simulink model "power_simulation2022a"  (R2022a)
settings: Solver=VariableStepAuto  StartTime=0.0  StopTime=600  RelTol=1e-3
values from neighbouring files (symbols this model uses):
  Ts = 5E-6    (= 5e-06)    [motor_variables.m]
undefined symbols (not defined in the file or in its folder): g_ft, sigbuilder_block
libraries: fl_lib x21, nesl_utility x11, ee_lib x4, sdl_lib x2
settings Model: Creator=OADEBAJO  LastModifiedBy=OADEBAJO

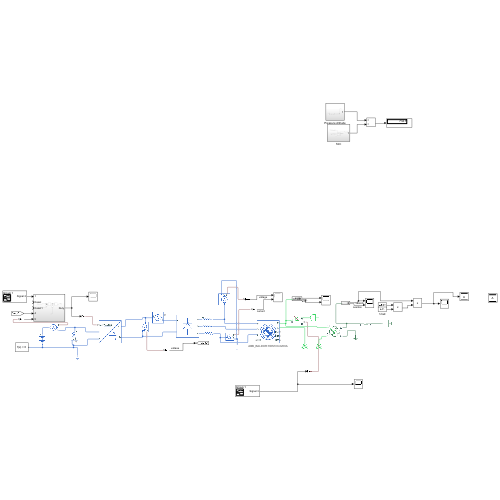
[thumbnail: Simulink's stored preview of the top-level diagram]
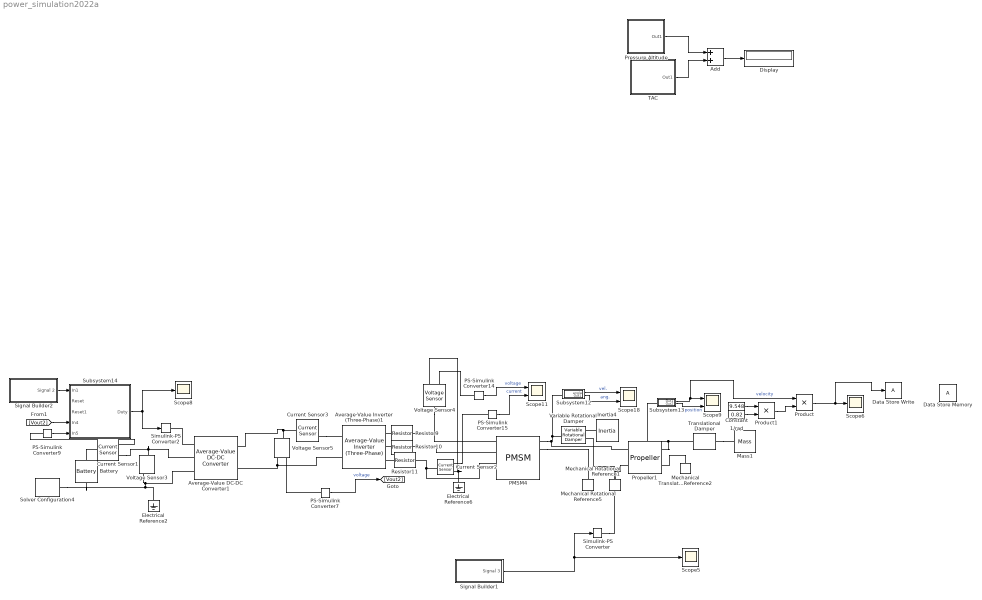
== system power_simulation2022a ==
  1/rad : Constant  Value=0.82
  Add : Sum
  Average-Value Inverter (Three-Phase)1 : ee_lib/Semiconductors & Converters/Converters/Average-Value Inverter (Three-Phase)  port_option=ee.enum.threePhasePort.expanded  FRated=60 Hz  PhaseShift=60 deg  voltage_ratio=sqrt(6) / pi  Pfixed=1e3 W  v_on=100 V  v_off=75 V
      settings: SourceProductBaseCode=PS  InternalSimscapePortConfiguration="{\"Bottom\":[],\"Left\":[{\"id\":\"p\",\"label\":\"+\",\"type\":\"foundation.electrical.electrical\"},{\"id\":\"n\",\"label\":\"-\",\"type\":\"foundation.electrical.electrical\"}],\"Right\":[{\"id\":\"a\",\"label\":\"a\",\"type\":\"foundation.electrical.electrical\"},{\"id\":\"b\",\"label\":\"b\",\"type\":\"foundation.electrical.electrical\"},{\"id\":\"c\",\"label\":\"c\",\"type\":\"foundation.electrical.electrical\"}],\"Top\":[]}"
  Average-Value DC-DC Converter1 : ee_lib/Semiconductors & Converters/Converters/Average-Value DC-DC Converter  control_option=ee.enum.converters.controlinput.dutycycle  converter_type=ee.enum.converters.dcdctype.buckboost  efficiency_option=ee.enum.converters.efficiency.constant  efficiency_fixed=95  i_vec=[0, 2, 5] A  efficiency_vec=[90, 95, 98]
      settings: SourceProductBaseCode=PS  InternalSimscapePortConfiguration="{\"Bottom\":[],\"Left\":[{\"id\":\"DutyCycle\",\"label\":\"DutyCycle\",\"type\":\"input\"},{\"id\":\"p1\",\"label\":\"1+\",\"type\":\"foundation.electrical.electrical\"},{\"id\":\"n1\",\"label\":\"1-\",\"type\":\"foundation.electrical.electrical\"}],\"Right\":[{\"id\":\"p2\",\"label\":\"2+\",\"type\":\"foundation.electrical.electrical\"},{\"id\":\"n2\",\"label\":\"2-\",\"type\":\"foundation.electrical.electrical\"}],\"Top\":[]}"
  Battery : ee_lib/Sources/Battery  Vnom=300 V  prm_dir=ee.enum.batterybasic.prm_dir.disabled  R1_dis=2 Ohm  R1_ch=2 Ohm  R1=0.001 Ohm  prm_AH=ee.enum.batterybasic.prm_AH.finite  AH=50 A*hr  V1=11.5 V  AH1=25 A*hr  prm_R2=ee.enum.batterybasic.prm_R2.disabled  R2=2000 Ohm  prm_dyn=ee.enum.batterybasic.prm_dyn.off  Rp1=0.005 Ohm  tau1=30 s  Rp2=0.005 Ohm  tau2=30 s  Rp3=0.005 Ohm  tau3=30 s  Rp4=0.005 Ohm  tau4=30 s  Rp5=0.005 Ohm  tau5=30 s  prm_fade=ee.enum.batterybasic.prm_fade.disabled  N_fade=100  AH_fade=45 A*hr  R1_fade=2.02 Ohm  R1_ch_fade=2.02 Ohm  V1_fade=10.35 V  prm_age=ee.enum.batterybasic.prm_age.disabled  prm_age_OCV=ee.enum.batterybasic.prm_age_OCV.OCV  OCV_age=0.9  SOC_age=60  delta_time_age_vec=[0] d  temperature_age_vec=[273] K  OCV_scaling_age=2.2134e6  OCV_offset_age=1.632e6  temp_exp_age=0.515833569 V  t_exp_age=0.75  i_specify=off  i_priority=None  i=0 A  i_nominal_specify=off  i_nominal_unit=A  i_nominal_value=1  v_specify=off  v_priority=None  v=0 V  v_nominal_specify=off  v_nominal_unit=V  v_nominal_value=1  charge_specify=off  charge_priority=High  charge=50 A*hr  charge_nominal_specify=off  charge_nominal_unit=A*hr  charge_nominal_value=1  num_cycles_specify=off  num_cycles_priority=High  num_cycles=0  num_cycles_nominal_specify=off  num_cycles_nominal_unit=1  num_cycles_nominal_value=1  Tmeas=298.15 K  Tmeas_age=298.15 K  Vnom_T2=12 V  R1_T2=2.2 Ohm  R1_T2_dis=2.2 Ohm  R1_T2_ch=2.2 Ohm  V1_T2=11.4 V  R2_T2=2200 Ohm  Rp1_T2=0.005 Ohm  tau1_T2=30 s  Rp2_T2=0.005 Ohm  tau2_T2=30 s  Rp3_T2=0.005 Ohm  tau3_T2=30 s  Rp4_T2=0.005 Ohm  tau4_T2=30 s  Rp5_T2=0.005 Ohm  tau5_T2=30 s  Tmeas2=273.15 K  thermal_mass=30000 J/K  temperature_specify=off  temperature_priority=High  temperature=298.15 K  temperature_nominal_specify=off  temperature_nominal_unit=K  temperature_nominal_value=1
  Constant : Constant  Value=9.548
  Current Sensor1 : fl_lib/Electrical/Electrical Sensors/Current Sensor
      settings: SourceProductBaseCode=PW,SS,VE
  Current Sensor2 : fl_lib/Electrical/Electrical Sensors/Current Sensor
      settings: SourceProductBaseCode=PW,SS,VE
  Current Sensor3 : fl_lib/Electrical/Electrical Sensors/Current Sensor
      settings: SourceProductBaseCode=PW,SS,VE
  Data Store Memory : DataStoreMemory  WriteAfterWriteMsg=warning  ShowAdditionalParam=off
  Data Store Write : DataStoreWrite  IndexOptions=Index vector (dialog)  Indices=1  OutputSizes=1
  Display : Display
  Electrical Reference2 : fl_lib/Electrical/Electrical Elements/Electrical Reference
      settings: SourceProductBaseCode=PW,SS,VE
  Electrical Reference6 : fl_lib/Electrical/Electrical Elements/Electrical Reference
      settings: SourceProductBaseCode=PW,SS,VE
  Inertia4 : fl_lib/Mechanical/Rotational Elements/Inertia  inertia=0.01 kg*m^2  num_ports=foundation.enum.numPorts2.one  w_specify=off  w_priority=High  w=0 rad/s  w_nominal_specify=off  w_nominal_unit=rad/s  w_nominal_value=1  t_specify=off  t_priority=None  t=0 N*m  t_nominal_specify=off  t_nominal_unit=N*m  t_nominal_value=1
      settings: SourceProductBaseCode=PW,SS,VE
  Mass1 : fl_lib/Mechanical/Translational Elements/Mass  mass=6 kg  num_ports=foundation.enum.numPorts2.one  v_specify=off  v_priority=High  v=0 m/s  v_nominal_specify=off  v_nominal_unit=m/s  v_nominal_value=1  f_specify=off  f_priority=None  f=0 N  f_nominal_specify=off  f_nominal_unit=N  f_nominal_value=1
      settings: SourceProductBaseCode=PW,SS,VE
  Mechanical Rotational Reference1 : fl_lib/Mechanical/Rotational Elements/Mechanical Rotational Reference
      settings: SourceProductBaseCode=PW,SS,VE
  Mechanical Rotational Reference5 : fl_lib/Mechanical/Rotational Elements/Mechanical Rotational Reference
      settings: SourceProductBaseCode=PW,SS,VE
  Mechanical Translational Reference2 : fl_lib/Mechanical/Translational Elements/Mechanical Translational Reference
      settings: SourceProductBaseCode=PW,SS,VE
  PMSM4 : ee_lib/Electromechanical/Permanent Magnet/PMSM  Tag={'toolbox/physmod/elec/library/m/ee_lib_parts';'Electromechanical/Permanent_Magnet/PMSM/ABB_BALDOR/HDS100_0206A.xml'}  port_option=ee.enum.threePhasePort.expanded  winding_type=ee.enum.statorconnection.wye  machine_param=ee.enum.pmsm.parameterization.constant  nPolePairs=5  pmflux_param=ee.enum.pmflux.fluxlinkage  pm_flux_linkage=0.0686133185085635 Wb  torque_constant=0.343066592542818 N*m/A  back_emf_constant=0.343066592542818 V/(rad/s)  stator_param=ee.enum.statorparam.LdLqL0  Ld=0.00855 H  Lq=0.00855 H  idVec=[-200 0 200] % Parameter not set A  iqVec=[-200 0 200] % Parameter not set A  LdMatrix=[0.0002 0.0002 0.0002;0.0002 0.0002 0.0002;0.0002 0.0002 0.0002] % Parameter not set H  LqMatrix=[0.0002 0.0002 0.0002;0.0002 0.0002 0.0002;0.0002 0.0002 0.0002] % Parameter not set H  PmMatrix=[0.1 0.1 0.1;0.1 0.1 0.1;0.1 0.1 0.1] Wb  ktMatrix=[0.18 0.18 0.18;0.18 0.18 0.18;0.18 0.18 0.18] N*m/A  keMatrix=[0.18 0.18 0.18;0.18 0.18 0.18;0.18 0.18 0.18] % Parameter not set V/(rad/s)  L0=[] % Parameter not set H  Ls=0.0002 H  Lm=-2e-05 H  Ms=2e-05 H  Rs=1.46 Ohm  zero_sequence=ee.enum.park.zerosequence.exclude  axes_param=ee.enum.rotorangle.daxis  loss_param=ee.enum.ironloss.none  losses_oc=[0 0 0] % Parameter not set W  losses_sc=[0 0 0] % Parameter not set W  f_losses=60 % Parameter not set Hz  Isc_losses=95 % Parameter not set A  J=7.6e-05 kg*m^2  lam=0 % Parameter not set N*m/(rad/s)  i_d_specify=off  i_d_priority=None  i_d=0 A  i_d_nominal_specify=off  i_d_nominal_unit=A  i_d_nominal_value=1  i_q_specify=off  i_q_priority=None  i_q=0 A  i_q_nominal_specify=off  i_q_nominal_unit=A  i_q_nominal_value=1  torque_specify=off  torque_priority=None  torque=0 N*m  torque_nominal_specify=off  torque_nominal_unit=N*m  torque_nominal_value=1  angular_velocity_specify=off  angular_velocity_priority=High  angular_velocity=0 rpm  angular_velocity_nominal_specify=off  angular_velocity_nominal_unit=rpm  angular_velocity_nominal_value=1  angular_position_specify=off  angular_position_priority=High  angular_position=0 deg  angular_position_nominal_specify=off  angular_position_nominal_unit=deg  angular_position_nominal_value=1  alpha=3.93e-3 1/K  alpha_flux=-0.001 1/K  Tmeas=298.15 K  stator_thermal_mass=100 J/K  rotor_thermal_mass=200 J/K  Rm_percent_rotor=90  Rd_percent_rotor=30  temperatureA_specify=off  temperatureA_priority=High  temperatureA=25 degC  temperatureA_nominal_specify=off  temperatureA_nominal_unit=degC  temperatureA_nominal_value=1  temperatureB_specify=off  temperatureB_priority=High  temperatureB=25 degC  temperatureB_nominal_specify=off  temperatureB_nominal_unit=degC  temperatureB_nominal_value=1  temperatureC_specify=off  temperatureC_priority=High  temperatureC=25 degC  temperatureC_nominal_specify=off  temperatureC_nominal_unit=degC  temperatureC_nominal_value=1  temperatureR_specify=off  temperatureR_priority=High  temperatureR=25 degC  temperatureR_nominal_specify=off  temperatureR_nominal_unit=degC  temperatureR_nominal_value=1
      settings: AttributesFormatString=ABB_BALDOR:HDS100-0206A  InternalSimscapePortConfiguration="{\"Bottom\":[],\"Left\":[{\"id\":\"a\",\"label\":\"a\",\"type\":\"foundation.electrical.electrical\"},{\"id\":\"b\",\"label\":\"b\",\"type\":\"foundation.electrical.electrical\"},{\"id\":\"c\",\"label\":\"c\",\"type\":\"foundation.electrical.electrical\"},{\"id\":\"HR\",\"label\":\"HR\",\"type\":\"foundation.thermal.thermal\"}],\"Right\":[{\"id\":\"R\",\"label\":\"R\",\"type\":\"foundation.mechanical.rotational.rotational\"},{\"id\":\"C\",\"label\":\"C\",\"type\":\"foundation.mechanical.rotational.rotational\"},{\"id\":\"HA\",\"label\":\"HA\",\"type\":\"foundation.thermal.thermal\"},{\"id\":\"HB\",\"label\":\"HB\",\"type\":\"foundation.thermal.thermal\"},{\"id\":\"HC\",\"label\":\"HC\",\"type\":\"foundation.thermal.thermal\"}],\"Top\":[]}"
  PS-Simulink Converter14 : nesl_utility/PS-Simulink Converter  PhysicalDomain=network_engine_domain  SubClassName=ps_output  LeftPortType=input  RightPortType=output  PseudoPeriodic=off  Frequencies=[]  VectorFormat=inherit  Unit=inherit  AffineConversion=off
      settings: SourceProductBaseCode=SS,PW,VE
  PS-Simulink Converter15 : nesl_utility/PS-Simulink Converter  PhysicalDomain=network_engine_domain  SubClassName=ps_output  LeftPortType=input  RightPortType=output  PseudoPeriodic=off  Frequencies=[]  VectorFormat=inherit  Unit=inherit  AffineConversion=off
      settings: SourceProductBaseCode=SS,PW,VE
  PS-Simulink Converter7 : nesl_utility/PS-Simulink Converter  PhysicalDomain=network_engine_domain  SubClassName=ps_output  LeftPortType=input  RightPortType=output  PseudoPeriodic=off  Frequencies=[]  VectorFormat=inherit  Unit=inherit  AffineConversion=off
      settings: SourceProductBaseCode=SS,PW,VE
  PS-Simulink Converter9 : nesl_utility/PS-Simulink Converter  PhysicalDomain=network_engine_domain  SubClassName=ps_output  LeftPortType=input  RightPortType=output  PseudoPeriodic=off  Frequencies=[]  VectorFormat=1-D array  Unit=A  AffineConversion=off
      settings: SourceProductBaseCode=SS,PW,VE
  Pressure Altitude : Subsystem
  Product : Product
  Product1 : Product
  Propeller1 : sdl_lib/Engines & Motors/Propeller  parameterization=sdl.enum.PropellerParameterization.Constant  pitch_type=foundation.enum.constant_controlled.constant  D=0.2 m  kt_const=0.25  kq_const=0.05  kt_poly_fixed=[.063, -.19, -.25, .37]  kq_poly_fixed=[.0043, -.021, -.03, .05]  pitch_ratio_TLU=[-.5, .5, .7, .9, 1.1, 1.4]  kt_poly_TLU=[.04, -.1, -.24, .12; .118, -.24, -.24, .19; .082, -.21, -.25, .28; .063, -.19, -.25, .37; .055, -.17, -.25, .45; .064, -.21, -.19, .55]  kq_poly_TLU=[.02, -.06, -.02, .02; .04, -.034, -.016, .018; .0076, -.02, -.023, .031; .0043, -.021, -.03, .05; .0047, -.024, -.036, .073; .0045, -.025, -.044, .11]  J_tab_TLU=[0, .3, .5, .7, .9, 1.2, 1.5]  kt_tab_fixed=[.37, .28, .21, .12, .033, -.098, -.23]  kq_tab_fixed=[.049, .039, .03, .02, .0096, -.0093, -.028]  kt_tab_TLU=[.12, .04, -.02, -.083, -.15, -.24, -.33; .19, .1, .029, -.047, -.12, -.23, -.35; .28, .19, .12, .032, -.054, -.18, -.31; .37, .28, .21, .12, .033, -.098, -.23; .45, .36, .29, .21, .13, -.0057, -.16; .54, .47, .41, .33, .25, .13, .0029]  kq_tab_TLU=[.02, .0091, -.0025, -.017, -.032, -.056, -.078; .017, .011, .006, .0009, -.0041, -.012, -.019; .03, .022, .015, .0074, -.0008, -.013, -.026; .049, .039, .03, .02, .0096, -.0093, -.028; .072, .06, .05, .038, .025, .0042, -.015; .11, .097, .085, .071, .057, .033, .0065]  interp_method=simscape.enum.interpolation.linear  extrap_method=simscape.enum.extrapolation.linear  density_spec=foundation.enum.constant_variable.constant  rho=1000 kg/m^3  translational_ports=sdl.enum.ConnectionType.Conserving  wake_fraction=0.2  efficiency_sensor=simscape.enum.onoff.off  n_thr=0.001 Hz  k_thr=0.001  operation_check=simscape.enum.assert.action.warn  w_specify=off  w_priority=None  w=0 rad/s  w_nominal_specify=off  w_nominal_unit=rad/s  w_nominal_value=1  Q_specify=off  Q_priority=None  Q=0 N*m  Q_nominal_specify=off  Q_nominal_unit=N*m  Q_nominal_value=1  v_specify=off  v_priority=None  v=0 m/s  v_nominal_specify=off  v_nominal_unit=m/s  v_nominal_value=1  thrust_specify=off  thrust_priority=None  thrust=0 N  thrust_nominal_specify=off  thrust_nominal_unit=N  thrust_nominal_value=1
      settings: SourceProductBaseCode=LD  InternalSimscapePortConfiguration="{\"Bottom\":[],\"Left\":[{\"id\":\"R1\",\"label\":\"R1\",\"type\":\"foundation.mechanical.rotational.rotational\"},{\"id\":\"C1\",\"label\":\"C1\",\"type\":\"foundation.mechanical.rotational.rotational\"}],\"Right\":[{\"id\":\"R2\",\"label\":\"R2\",\"type\":\"foundation.mechanical.translational.translational\"},{\"id\":\"C2\",\"label\":\"C2\",\"type\":\"foundation.mechanical.translational.translational\"}],\"Top\":[]}"
  Resistor10 : fl_lib/Electrical/Electrical Elements/Resistor  R=10 Ohm  i_specify=off  i_priority=None  i=0 A  i_nominal_specify=off  i_nominal_unit=A  i_nominal_value=1  v_specify=off  v_priority=None  v=0 V  v_nominal_specify=off  v_nominal_unit=V  v_nominal_value=1
      settings: SourceProductBaseCode=PW,SS,VE
  Resistor11 : fl_lib/Electrical/Electrical Elements/Resistor  R=10 Ohm  i_specify=off  i_priority=None  i=0 A  i_nominal_specify=off  i_nominal_unit=A  i_nominal_value=1  v_specify=off  v_priority=None  v=0 V  v_nominal_specify=off  v_nominal_unit=V  v_nominal_value=1
      settings: SourceProductBaseCode=PW,SS,VE
  Resistor9 : fl_lib/Electrical/Electrical Elements/Resistor  R=10 Ohm  i_specify=off  i_priority=None  i=0 A  i_nominal_specify=off  i_nominal_unit=A  i_nominal_value=1  v_specify=off  v_priority=None  v=0 V  v_nominal_specify=off  v_nominal_unit=V  v_nominal_value=1
      settings: SourceProductBaseCode=PW,SS,VE
  Scope11 : Scope  NumInputPorts=2
  Scope18 : Scope  NumInputPorts=2
  Scope5 : Scope
  Scope6 : Scope
  Scope8 : Scope
  Scope9 : Scope  NumInputPorts=2
  Signal Builder1 : Subsystem  Tag=STV Subsys  LoadFcn=sigbuilder_block('load');  StartFcn=sigbuilder_block('start');  StopFcn=sigbuilder_block('stop');  ClipboardFcn=sigbuilder_block('clipboard');  mask(Sigbuilder block){tuvar=[0:10]}
      mask help: Simulink:masks:SigbuilderBlock_MD
      mask init:
      | if ~strcmp(get_param(bdroot(gcbh),'SimulationStatus'),'stopped') tuvar = sigbuilder_block('maskInit'); end
      settings: CopyFcn=sigbuilder_block('copy');  DeleteFcn=sigbuilder_block('delete');  ModelCloseFcn=sigbuilder_block('modelClose');  PreSaveFcn=sigbuilder_block('preSave');  PauseFcn=sigbuilder_block('pause');  ContinueFcn=sigbuilder_block('continue');  NameChangeFcn=sigbuilder_block('namechange');  OpenFcn=sigbuilder_block('open',[255.75 99 836.25 501.75 ]);  CloseFcn=sigbuilder_block('close');
      mask Display: plot(0, 0, 100, 100,[2, 2, 32, 32, 2], [68, 8, 8, 68, 68],[32, 2], [38, 38], [32, 19, 2],[53, 60, 44], [32, 17, 17, 2],[16, 16, 31, 31]);txt = getActiveGroup(gcbh);text(2, 100, txt,'verticalAlignment', 'top');
  Signal Builder2 : Subsystem  Tag=STV Subsys  LoadFcn=sigbuilder_block('load');  StartFcn=sigbuilder_block('start');  StopFcn=sigbuilder_block('stop');  ClipboardFcn=sigbuilder_block('clipboard');  mask(Sigbuilder block){tuvar=[0:10]}
      mask help: Simulink:masks:SigbuilderBlock_MD
      mask init:
      | if ~strcmp(get_param(bdroot(gcbh),'SimulationStatus'),'stopped') tuvar = sigbuilder_block('maskInit'); end
      settings: CopyFcn=sigbuilder_block('copy');  DeleteFcn=sigbuilder_block('delete');  ModelCloseFcn=sigbuilder_block('modelClose');  PreSaveFcn=sigbuilder_block('preSave');  PauseFcn=sigbuilder_block('pause');  ContinueFcn=sigbuilder_block('continue');  NameChangeFcn=sigbuilder_block('namechange');  OpenFcn=sigbuilder_block('open',[255.75 99 836.25 501.75 ]);  CloseFcn=sigbuilder_block('close');
      mask Display: plot(0, 0, 100, 100,[2, 2, 32, 32, 2], [68, 8, 8, 68, 68],[32, 2], [38, 38], [32, 19, 2],[53, 60, 44], [32, 17, 17, 2],[16, 16, 31, 31]);txt = getActiveGroup(gcbh);text(2, 100, txt,'verticalAlignment', 'top');
  Simulink-PS Converter : nesl_utility/Simulink-PS Converter  PhysicalDomain=network_engine_domain  SubClassName=ps_input  LeftPortType=input  RightPortType=output  PseudoPeriodic=off  Frequencies=[]  NoiseDistribution=none  NoiseParameters=[]  Unit=1  AffineConversion=off  FilteringAndDerivatives=provide  SimscapeFilterOrder=1  InputFilterTimeConstant=0.001  UdotUserProvided=0
      settings: SourceProductBaseCode=SS,PW,VE
  Simulink-PS Converter2 : nesl_utility/Simulink-PS Converter  PhysicalDomain=network_engine_domain  SubClassName=ps_input  LeftPortType=input  RightPortType=output  PseudoPeriodic=off  Frequencies=[]  NoiseDistribution=none  NoiseParameters=[]  Unit=1  AffineConversion=off  FilteringAndDerivatives=provide  SimscapeFilterOrder=1  InputFilterTimeConstant=0.001  UdotUserProvided=0
      settings: SourceProductBaseCode=SS,PW,VE
  Solver Configuration4 : nesl_utility/Solver Configuration  PhysicalDomain=network_engine_domain  SubClassName=solver  LeftPortType=input  RightPortType=generic  Tones=[]  Harmonics=[]  SimulateNoise=off  Profile=off  UseLocalSampling=off  EnableSwitchedLinearOptims=on  FrequencyDomain=off  UseCCode=off  RelTol=0.001  AbsTol=1e-06  MinStep=1e-09  ToWorkspace=off  RevertToSquareIcSolve=off  NumHomotopyIterations=100  PhasorMode=off  PhasorModeNumHarmonics=1  IndexReductionMethod=DerivativeReplacement  DoDC=off  ResidualTolerance=1e-3  UseLocalSolver=on  LocalSolverChoice=NE_BACKWARD_EULER_ADVANCER  LocalSolverSampleTime=1e-4  DoFixedCost=on  MaxNonlinIter=3  MaxModeIter=2  ComputeImpulses=off  ImpulseIterations=2  LinearAlgebra=auto  LinearAlgebraNumThread=0  EquationFormulation=NE_TIME_EF  DelaysMemoryBudget=1024  AutomaticFiltering=off  FilteringTimeConstant=0.001  PartitionStorageMethod=AS_NEEDED  PartitionMemoryBudget=1024  PartitionMethod=FAST
      settings: SourceProductBaseCode=SS,PW,VE
  Subsystem12 : Subsystem
  Subsystem13 : Subsystem
  Subsystem14 : Subsystem
  TAC : Subsystem
  Translational Damper : fl_lib/Mechanical/Translational Elements/Translational Damper  D=100 N*s/m  v_specify=off  v_priority=None  v=0 m/s  v_nominal_specify=off  v_nominal_unit=m/s  v_nominal_value=1  f_specify=off  f_priority=None  f=0 N  f_nominal_specify=off  f_nominal_unit=N  f_nominal_value=1
      settings: SourceProductBaseCode=PW,SS,VE
  Variable Rotational Damper : sdl_lib/Couplings & Drives/Springs & Dampers/Variable Rotational Damper  Bmin=0 N*m*s/rad
      settings: SourceProductBaseCode=LD  InternalSimscapePortConfiguration="{\"Bottom\":[],\"Left\":[{\"id\":\"B\",\"label\":\"B\",\"type\":\"input\"},{\"id\":\"R\",\"label\":\"R\",\"type\":\"foundation.mechanical.rotational.rotational\"}],\"Right\":[{\"id\":\"C\",\"label\":\"C\",\"type\":\"foundation.mechanical.rotational.rotational\"}],\"Top\":[]}"
  Voltage Sensor3 : fl_lib/Electrical/Electrical Sensors/Voltage Sensor
      settings: SourceProductBaseCode=PW,SS,VE
  Voltage Sensor4 : fl_lib/Electrical/Electrical Sensors/Voltage Sensor
      settings: SourceProductBaseCode=PW,SS,VE
  Voltage Sensor5 : fl_lib/Electrical/Electrical Sensors/Voltage Sensor
      settings: SourceProductBaseCode=PW,SS,VE
  wires:
  Pressure Altitude/1(Out1) -> Add/1
  TAC/1(Out1) -> Add/2
  Add/1 -> Display/1
  PS-Simulink Converter7/1 -> [Vout2]  "voltage"
  [Vout2] -> Subsystem14/4(In4)
  Subsystem12/1(angle) -> Scope18/1  "vel."
  PS-Simulink Converter9/1 -> Subsystem14/5(In5)
  Subsystem12/2(Out1) -> Scope18/2  "ang."
  Subsystem14/1(Duty) -> Simulink-PS Converter2/1, Scope8/1
  Subsystem13/2(Out2) -> Scope9/2  "position"
  Subsystem13/1(Out1) -> Product/1, Scope9/1  "velocity"
  Signal Builder2/1(Signal 2) -> Subsystem14/1(In1)
  Signal Builder1/1(Signal 3) -> Simulink-PS Converter/1, Scope5/1
  Constant/1 -> Product1/1
  1/rad/1 -> Product1/2
  Product1/1 -> Product/2
  Product/1 -> Data Store Write/1, Scope6/1
  PS-Simulink Converter14/1 -> Scope11/1  "voltage"
  PS-Simulink Converter15/1 -> Scope11/2  "current"
  connections:
  Voltage Sensor3/RConn2 -- Average-Value DC-DC Converter1/LConn3 -- Electrical Reference2/LConn1 -- Battery/RConn1 -- Solver Configuration4/RConn1
  PMSM4/RConn1 -- Propeller1/LConn1 -- Variable Rotational Damper/RConn1 -- Subsystem12/LConn1
  Translational Damper/RConn1 -- Propeller1/RConn1 -- Subsystem13/LConn1
  Current Sensor1/RConn2 -- Average-Value DC-DC Converter1/LConn2 -- Voltage Sensor3/LConn1
  Current Sensor3/LConn1 -- Average-Value DC-DC Converter1/RConn1 -- Voltage Sensor5/LConn1
  Average-Value Inverter (Three-Phase)1/LConn2 -- Average-Value DC-DC Converter1/RConn2 -- Voltage Sensor5/RConn2
  Simulink-PS Converter/RConn1 -- Variable Rotational Damper/LConn1
  Average-Value Inverter (Three-Phase)1/RConn3 -- Resistor11/LConn1
  Resistor10/RConn1 -- PMSM4/LConn2
  Current Sensor1/LConn1 -- Battery/LConn1
  PS-Simulink Converter9/LConn1 -- Current Sensor1/RConn1
  Translational Damper/LConn1 -- Mass1/LConn1
  Average-Value DC-DC Converter1/LConn1 -- Simulink-PS Converter2/RConn1
  Current Sensor2/LConn1 -- Resistor11/RConn1 -- PMSM4/LConn3
  Resistor9/RConn1 -- Voltage Sensor4/LConn1 -- PMSM4/LConn1
  Current Sensor3/RConn2 -- Average-Value Inverter (Three-Phase)1/LConn1
  Propeller1/RConn2 -- Mechanical Translational Reference2/LConn1
  Average-Value Inverter (Three-Phase)1/RConn2 -- Resistor10/LConn1
  Inertia4/LConn1 -- Variable Rotational Damper/LConn2
  Voltage Sensor5/RConn1 -- PS-Simulink Converter7/LConn1
  Average-Value Inverter (Three-Phase)1/RConn1 -- Resistor9/LConn1
  PMSM4/RConn2 -- Mechanical Rotational Reference5/LConn1
  Current Sensor2/RConn1 -- PS-Simulink Converter15/LConn1
  Current Sensor2/RConn2 -- Voltage Sensor4/RConn2 -- Electrical Reference6/LConn1
  Voltage Sensor4/RConn1 -- PS-Simulink Converter14/LConn1
  Propeller1/LConn2 -- Mechanical Rotational Reference1/LConn1

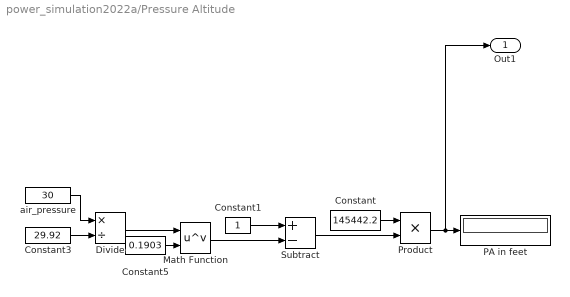
== system power_simulation2022a/Pressure Altitude ==
  Constant : Constant  Value=145442.2
  Constant1 : Constant
  Constant3 : Constant  Value=29.92
  Constant5 : Constant  Value=0.1903
  Divide : Product  Inputs=*/
  Math Function : Math  Operator=pow  SignedPower=on
  PA in feet : Display
  Product : Product
  Subtract : Sum  Inputs=+-
  air_pressure : Constant  Value=30
  Out1 : Outport
  wires:
  Constant5/1 -> Math Function/2
  Math Function/1 -> Subtract/2
  Constant/1 -> Product/1
  Product/1 -> Out1/1, PA in feet/1
  Divide/1 -> Math Function/1
  air_pressure/1 -> Divide/1
  Constant3/1 -> Divide/2
  Constant1/1 -> Subtract/1
  Subtract/1 -> Product/2

== system power_simulation2022a/Signal Builder1 ==
  Demux : Demux  Tag=STV Demux  Outputs=1
      settings: DisplayOption=none
  FromWs : FromWorkspace  Tag=STV FromWs  VariableName=tuvar
      SigBuilderData=|
      | common.afterFinalStr = 'Extrapolate'
      | common.sampleTime = 0
      | dataSet.timeRange = [0 600]
      | dataSet.name = 'Group 1'
      | sbobj.Groups.Name = 'Group 1'
      | sbobj.Groups.Signals.Name = 'Signal 3'
      | sbobj.Groups.Signals.XData = [0 100 100 360 360 450 450 600]
      | sbobj.Groups.Signals.YData = [130 130 200 200 185 185 125 125]
      | sbobj.Groups.TimeRange = [0 600]
  Signal 3 : Outport  Tag=STV Outport
  wires:
  FromWs/1 -> Demux/1
  Demux/1 -> Signal 3/1

== system power_simulation2022a/Signal Builder2 ==
  Demux : Demux  Tag=STV Demux  Outputs=1
      settings: DisplayOption=none
  FromWs : FromWorkspace  Tag=STV FromWs  VariableName=tuvar
      SigBuilderData=|
      | common.afterFinalStr = 'Extrapolate'
      | common.sampleTime = 0
      | dataSet.timeRange = [0 3600]
      | dataSet.name = 'Group 1'
      | sbobj.Groups.Name = 'Group 1'
      | sbobj.Groups.Signals.Name = 'Signal 2'
      | sbobj.Groups.Signals.XData = [0 4 770 2500 2500 3600]
      | sbobj.Groups.Signals.YData = [279.5 280 280 280 279.9 280]
      | sbobj.Groups.TimeRange = [0 3600]
  Signal 2 : Outport  Tag=STV Outport
  wires:
  FromWs/1 -> Demux/1
  Demux/1 -> Signal 2/1

== system power_simulation2022a/Subsystem12 ==
  Ideal Rotational Motion Sensor4 : fl_lib/Mechanical/Mechanical Sensors/Ideal Rotational Motion Sensor  wrap_angle=simscape.enum.onoff.off  offset=0 rad
      settings: SourceProductBaseCode=PW,SS,VE
  Mechanical Rotational Reference : fl_lib/Mechanical/Rotational Elements/Mechanical Rotational Reference
      settings: SourceProductBaseCode=PW,SS,VE
  PS-Simulink Converter : nesl_utility/PS-Simulink Converter  PhysicalDomain=network_engine_domain  SubClassName=ps_output  LeftPortType=input  RightPortType=output  PseudoPeriodic=off  Frequencies=[]  VectorFormat=inherit  Unit=inherit  AffineConversion=off
      settings: SourceProductBaseCode=SS,PW,VE
  PS-Simulink Converter7 : nesl_utility/PS-Simulink Converter  PhysicalDomain=network_engine_domain  SubClassName=ps_output  LeftPortType=input  RightPortType=output  PseudoPeriodic=off  Frequencies=[]  VectorFormat=inherit  Unit=inherit  AffineConversion=off
      settings: SourceProductBaseCode=SS,PW,VE
  Conn3 : PMIOPort  Side=Left
  angle : Outport
  Out1 : Outport  Port=2
  wires:
  PS-Simulink Converter7/1 -> angle/1  "ang. velocity"
  PS-Simulink Converter/1 -> Out1/1
  connections:
  Ideal Rotational Motion Sensor4/RConn2 -- PS-Simulink Converter7/LConn1
  PS-Simulink Converter/LConn1 -- Ideal Rotational Motion Sensor4/RConn3
  Conn3/RConn1 -- Ideal Rotational Motion Sensor4/LConn1
  Ideal Rotational Motion Sensor4/RConn1 -- Mechanical Rotational Reference/LConn1

== system power_simulation2022a/Subsystem13 ==
  Ideal Translational Motion Sensor : fl_lib/Mechanical/Mechanical Sensors/Ideal Translational Motion Sensor  offset=0 m
      settings: SourceProductBaseCode=PW,SS,VE
  Mechanical Translational Reference : fl_lib/Mechanical/Translational Elements/Mechanical Translational Reference
      settings: SourceProductBaseCode=PW,SS,VE
  PS-Simulink Converter : nesl_utility/PS-Simulink Converter  PhysicalDomain=network_engine_domain  SubClassName=ps_output  LeftPortType=input  RightPortType=output  PseudoPeriodic=off  Frequencies=[]  VectorFormat=inherit  Unit=inherit  AffineConversion=off
      settings: SourceProductBaseCode=SS,PW,VE
  PS-Simulink Converter1 : nesl_utility/PS-Simulink Converter  PhysicalDomain=network_engine_domain  SubClassName=ps_output  LeftPortType=input  RightPortType=output  PseudoPeriodic=off  Frequencies=[]  VectorFormat=inherit  Unit=inherit  AffineConversion=off
      settings: SourceProductBaseCode=SS,PW,VE
  . : PMIOPort  Side=Left
  Out1 : Outport
  Out2 : Outport  Port=2
  wires:
  PS-Simulink Converter/1 -> Out1/1  "velocity"
  PS-Simulink Converter1/1 -> Out2/1  "position"
  connections:
  Ideal Translational Motion Sensor/LConn1 -- ./RConn1
  Ideal Translational Motion Sensor/RConn2 -- PS-Simulink Converter/LConn1
  Ideal Translational Motion Sensor/RConn3 -- PS-Simulink Converter1/LConn1
  Ideal Translational Motion Sensor/RConn1 -- Mechanical Translational Reference/LConn1

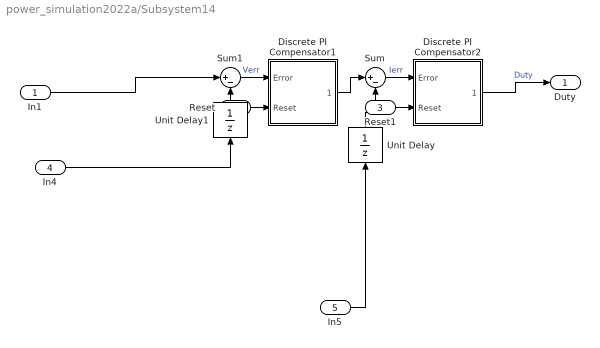
== system power_simulation2022a/Subsystem14 ==
  In1 : Inport
  Reset : Inport  Port=2
  Reset1 : Inport  Port=3
  In4 : Inport  Port=4
  In5 : Inport  Port=5
  Discrete PI Compensator1 : Subsystem  mask{Kp=2.593/10000, Ki=1496.8*1, Ts_PI=Ts, UpSat=35, LowSat=-35, Initial_Condition=0}
      mask prompts: Kp "Kp Value"; Ki "Ki Value"; Ts_PI "Sample Time"; UpSat "Saturation Upper Limit"; LowSat "Saturation Lower Limit"; Initial_Condition "Initial Condition"
      mask DialogControl DescTextVar Prompt: %<Discrete PI Compensator using trapezoidal approximation for integration with saturation and back-clamping.>
  Discrete PI Compensator2 : Subsystem  mask{Kp=0.31/100, Ki=4534.18/100, Ts_PI=Ts, UpSat=0.9, LowSat=0, Initial_Condition=0}
      mask prompts: Kp "Kp Value"; Ki "Ki Value"; Ts_PI "Sample Time"; UpSat "Saturation Upper Limit"; LowSat "Saturation Lower Limit"; Initial_Condition "Initial Condition"
      mask DialogControl DescTextVar Prompt: %<Discrete PI Compensator using trapezoidal approximation for integration with saturation and back-clamping.>
  Sum : Sum  Inputs=|+-
  Sum1 : Sum  Inputs=|+-
  Unit Delay : UnitDelay  SampleTime=-1  HasFrameUpgradeWarning=on
  Unit Delay1 : UnitDelay  SampleTime=-1  HasFrameUpgradeWarning=on
  Duty : Outport
  wires:
  Sum/1 -> Discrete PI Compensator2/1(Error)  "Ierr"
  Unit Delay/1 -> Sum/2
  Unit Delay1/1 -> Sum1/2
  Discrete PI Compensator2/1(Signal Out) -> Duty/1  "Duty"
  Sum1/1 -> Discrete PI Compensator1/1(Error)  "Verr"
  Discrete PI Compensator1/1(Signal Out) -> Sum/1
  In1/1 -> Sum1/1
  In4/1 -> Unit Delay1/1
  In5/1 -> Unit Delay/1
  Reset1/1 -> Discrete PI Compensator2/2(Reset)
  Reset/1 -> Discrete PI Compensator1/2(Reset)

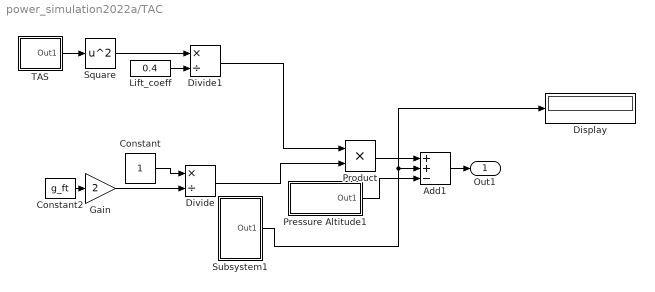
== system power_simulation2022a/TAC ==
  Add1 : Sum  Inputs=++-
  Constant : Constant
  Constant2 : Constant  Value=g_ft
  Display : Display
  Divide : Product  Inputs=*/
  Divide1 : Product  Inputs=*/
  Gain : Gain  Gain=2
  Lift_coeff : Constant  Value=0.4
  Pressure Altitude1 : Subsystem
  Product : Product
  Square : Math  Operator=square
  Subsystem1 : Subsystem
  TAS : Subsystem
  Out1 : Outport
  wires:
  Subsystem1/1(Out1) -> Display/1, Add1/2
  Pressure Altitude1/1(Out1) -> Add1/3
  Square/1 -> Divide1/1
  TAS/1(Out1) -> Square/1
  Constant/1 -> Divide/1
  Product/1 -> Add1/1
  Gain/1 -> Divide/2
  Divide1/1 -> Product/1
  Divide/1 -> Product/2
  Lift_coeff/1 -> Divide1/2
  Constant2/1 -> Gain/1
  Add1/1 -> Out1/1

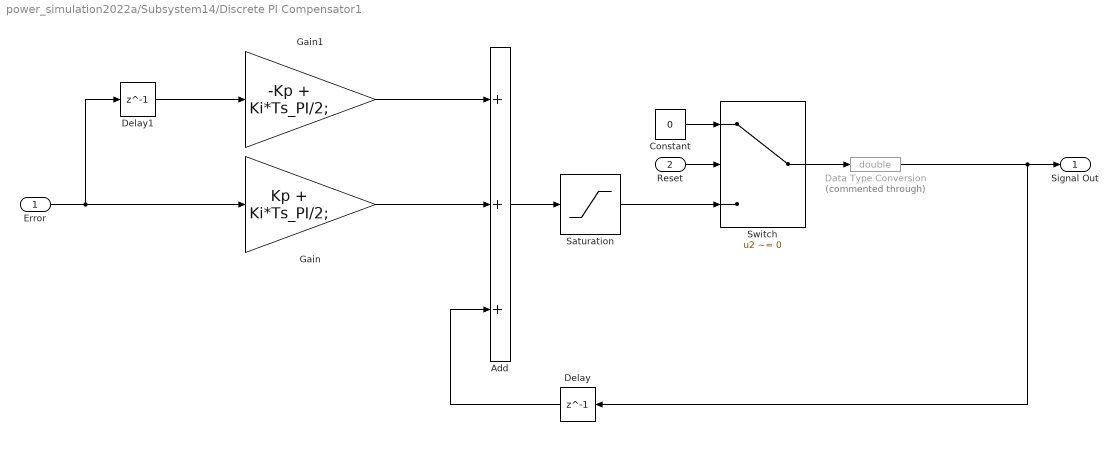
== system power_simulation2022a/Subsystem14/Discrete PI Compensator1 ==
  Error : Inport
  Reset : Inport  Port=2
  Add : Sum  Inputs=+++  AccumDataTypeStr=single
  Constant : Constant  Value=0
  Data Type Conversion : DataTypeConversion  Commented=through  OutDataTypeStr=double  SaturateOnIntegerOverflow=off  RndMeth=Floor
  Delay : Delay  DelayLength=1
  Delay1 : Delay  DelayLength=1  InitialCondition=Initial_Condition
  Gain : Gain  Gain=Kp + Ki*Ts_PI/2;
  Gain1 : Gain  Gain="-Kp +  Ki*Ts_PI/2;"
  Saturation : Saturate  UpperLimit=UpSat  LowerLimit=LowSat  OutDataTypeStr=single
  Switch : Switch  Criteria=u2 ~= 0  Threshold=0.5  SaturateOnIntegerOverflow=off  InputSameDT=off
  Signal Out : Outport
  wires:
  Data Type Conversion/1 -> Signal Out/1, Delay/1
  Constant/1 -> Switch/1
  Switch/1 -> Data Type Conversion/1
  Reset/1 -> Switch/2
  Saturation/1 -> Switch/3
  Gain1/1 -> Add/1
  Delay1/1 -> Gain1/1
  Gain/1 -> Add/2
  Delay/1 -> Add/3
  Error/1 -> Gain/1, Delay1/1
  Add/1 -> Saturation/1

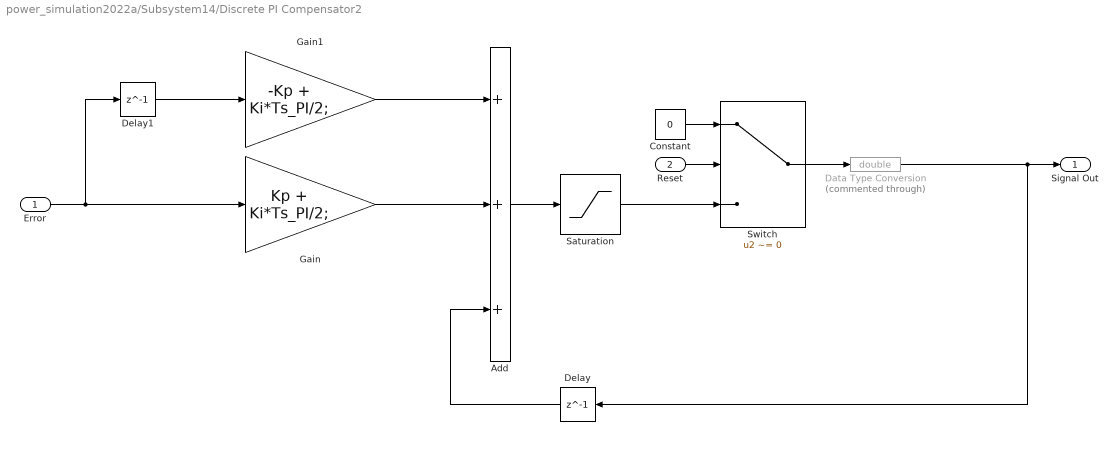
== system power_simulation2022a/Subsystem14/Discrete PI Compensator2 ==
  Error : Inport
  Reset : Inport  Port=2
  Add : Sum  Inputs=+++  AccumDataTypeStr=single
  Constant : Constant  Value=0
  Data Type Conversion : DataTypeConversion  Commented=through  OutDataTypeStr=double  SaturateOnIntegerOverflow=off  RndMeth=Floor
  Delay : Delay  DelayLength=1
  Delay1 : Delay  DelayLength=1  InitialCondition=Initial_Condition
  Gain : Gain  Gain=Kp + Ki*Ts_PI/2;
  Gain1 : Gain  Gain="-Kp +  Ki*Ts_PI/2;"
  Saturation : Saturate  UpperLimit=UpSat  LowerLimit=LowSat  OutDataTypeStr=single
  Switch : Switch  Criteria=u2 ~= 0  Threshold=0.5  SaturateOnIntegerOverflow=off  InputSameDT=off
  Signal Out : Outport
  wires:
  Add/1 -> Saturation/1
  Error/1 -> Delay1/1, Gain/1
  Delay/1 -> Add/3
  Gain/1 -> Add/2
  Delay1/1 -> Gain1/1
  Gain1/1 -> Add/1
  Saturation/1 -> Switch/3
  Reset/1 -> Switch/2
  Switch/1 -> Data Type Conversion/1
  Constant/1 -> Switch/1
  Data Type Conversion/1 -> Delay/1, Signal Out/1

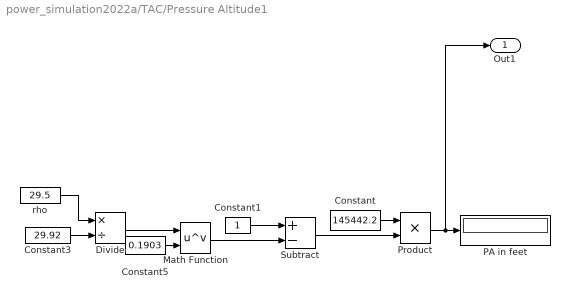
== system power_simulation2022a/TAC/Pressure Altitude1 ==
  Constant : Constant  Value=145442.2
  Constant1 : Constant
  Constant3 : Constant  Value=29.92
  Constant5 : Constant  Value=0.1903
  Divide : Product  Inputs=*/
  Math Function : Math  Operator=pow
  PA in feet : Display
  Product : Product
  Subtract : Sum  Inputs=+-
  rho : Constant  Value=29.5
  Out1 : Outport
  wires:
  Constant5/1 -> Math Function/2
  Math Function/1 -> Subtract/2
  Constant/1 -> Product/1
  Product/1 -> Out1/1, PA in feet/1
  Divide/1 -> Math Function/1
  rho/1 -> Divide/1
  Constant3/1 -> Divide/2
  Constant1/1 -> Subtract/1
  Subtract/1 -> Product/2

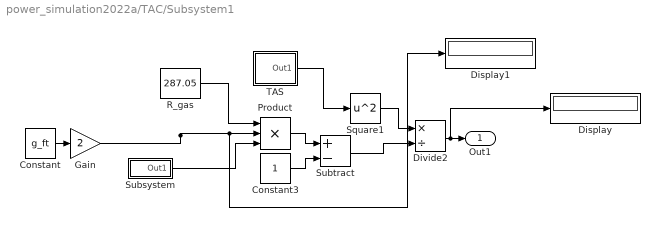
== system power_simulation2022a/TAC/Subsystem1 ==
  Constant : Constant  Value=g_ft
  Constant3 : Constant
  Display : Display
  Display1 : Display
  Divide2 : Product  Inputs=*/
  Gain : Gain  Gain=2
  Product : Product  Inputs=3
  R_gas : Constant  Value=287.05
  Square1 : Math  Operator=square
  Subsystem : Subsystem
  Subtract : Sum  Inputs=+-
  TAS : Subsystem
  Out1 : Outport
  wires:
  Product/1 -> Subtract/1
  Constant3/1 -> Subtract/2
  R_gas/1 -> Product/1
  Square1/1 -> Divide2/1
  TAS/1(Out1) -> Square1/1
  Gain/1 -> Display1/1, Product/2
  Constant/1 -> Gain/1
  Subsystem/1(Out1) -> Product/3
  Subtract/1 -> Divide2/2
  Divide2/1 -> Display/1, Out1/1

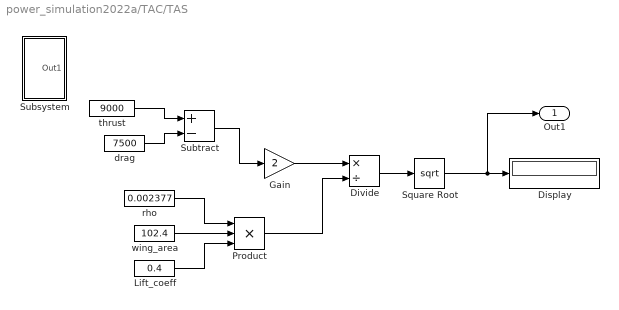
== system power_simulation2022a/TAC/TAS ==
  Display : Display
  Divide : Product  Inputs=*/
  Gain : Gain  Gain=2
  Lift_coeff : Constant  Value=0.4
  Product : Product  Inputs=3
  Square Root : Sqrt
  Subsystem : Subsystem
  Subtract : Sum  Inputs=+-
  drag : Constant  Value=7500
  rho : Constant  Value=0.002377
  thrust : Constant  Value=9000
  wing_area : Constant  Value=102.4
  Out1 : Outport
  wires:
  Divide/1 -> Square Root/1
  Product/1 -> Divide/2
  wing_area/1 -> Product/2
  Gain/1 -> Divide/1
  Subtract/1 -> Gain/1
  thrust/1 -> Subtract/1
  rho/1 -> Product/1
  Square Root/1 -> Display/1, Out1/1
  Lift_coeff/1 -> Product/3
  drag/1 -> Subtract/2

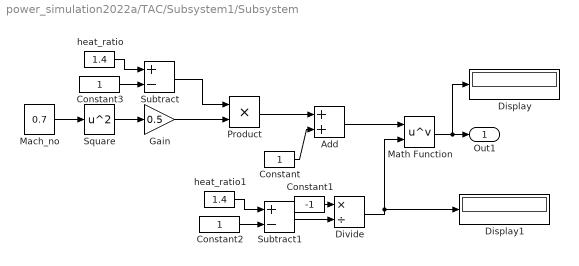
== system power_simulation2022a/TAC/Subsystem1/Subsystem ==
  Add : Sum
  Constant : Constant
  Constant1 : Constant  Value=-1
  Constant2 : Constant
  Constant3 : Constant
  Display : Display
  Display1 : Display
  Divide : Product  Inputs=*/
  Gain : Gain  Gain=0.5
  Mach_no : Constant  Value=0.7
  Math Function : Math  Operator=pow
  Product : Product
  Square : Math  Operator=square
  Subtract : Sum  Inputs=+-
  Subtract1 : Sum  Inputs=+-
  heat_ratio : Constant  Value=1.4
  heat_ratio1 : Constant  Value=1.4
  Out1 : Outport
  wires:
  Constant3/1 -> Subtract/2
  heat_ratio/1 -> Subtract/1
  Subtract/1 -> Product/1
  Mach_no/1 -> Square/1
  Square/1 -> Gain/1
  Gain/1 -> Product/2
  Product/1 -> Add/1
  Constant/1 -> Add/2
  Add/1 -> Math Function/1
  Constant2/1 -> Subtract1/2
  heat_ratio1/1 -> Subtract1/1
  Subtract1/1 -> Divide/2
  Constant1/1 -> Divide/1
  Divide/1 -> Math Function/2, Display1/1
  Math Function/1 -> Display/1, Out1/1

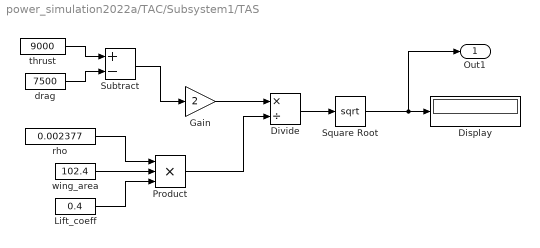
== system power_simulation2022a/TAC/Subsystem1/TAS ==
  Display : Display
  Divide : Product  Inputs=*/
  Gain : Gain  Gain=2
  Lift_coeff : Constant  Value=0.4
  Product : Product  Inputs=3
  Square Root : Sqrt
  Subtract : Sum  Inputs=+-
  drag : Constant  Value=7500
  rho : Constant  Value=0.002377
  thrust : Constant  Value=9000
  wing_area : Constant  Value=102.4
  Out1 : Outport
  wires:
  Divide/1 -> Square Root/1
  Product/1 -> Divide/2
  wing_area/1 -> Product/2
  Gain/1 -> Divide/1
  Subtract/1 -> Gain/1
  thrust/1 -> Subtract/1
  rho/1 -> Product/1
  Square Root/1 -> Out1/1, Display/1
  Lift_coeff/1 -> Product/3
  drag/1 -> Subtract/2

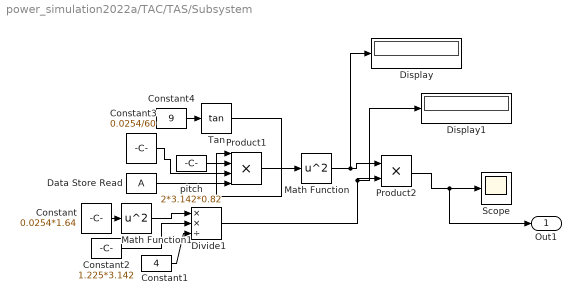
== system power_simulation2022a/TAC/TAS/Subsystem ==
  Constant : Constant  Value=0.0254*1.64
  Constant1 : Constant  Value=4
  Constant2 : Constant  Value=1.225*3.142
  Constant3 : Constant  Value=0.0254/60
  Constant4 : Constant  Value=9
  Data Store Read : DataStoreRead  IndexOptions=Index vector (dialog)  Indices=1  OutputSizes=1
  Display : Display
  Display1 : Display
  Divide1 : Product  Inputs=**/
  Math Function : Math  Operator=square
  Math Function1 : Math  Operator=square
  Product1 : Product  Inputs=4
  Product2 : Product
  Scope : Scope
  Tan : Trigonometry  Operator=tan
  pitch : Constant  Value=2*3.142*0.82
  Out1 : Outport
  wires:
  Math Function1/1 -> Divide1/1
  Constant2/1 -> Divide1/2
  pitch/1 -> Product1/2
  Constant/1 -> Math Function1/1
  Constant3/1 -> Product1/3
  Data Store Read/1 -> Product1/4
  Constant1/1 -> Divide1/3
  Tan/1 -> Product1/1
  Constant4/1 -> Tan/1
  Product1/1 -> Math Function/1
  Product2/1 -> Out1/1, Scope/1
  Divide1/1 -> Display1/1, Product2/2
  Math Function/1 -> Display/1, Product2/1
